simulink model "AbstractFuelControl_M3"  (R2015b)
settings: Solver=FixedStepAuto  StartTime=0.0  StopTime=simTime  RelTol=1e-3
undefined symbols (not defined in the file or in its folder): c1, c11, c12, c13, c14, c15, c16, c17, c18, c19, c2, c20, c21, c22, c23, c24, c25, c3, c4, c5, c6, c7, c8, c9, fault_time, measureTime, simTime, spec_num
settings Model: Creator=xjin  LastModifiedBy=potok
settings DataIOCC: ExternalInput=[simTime, en_speed]  LimitDataPoints=off  LoadExternalInput=on  SaveFormat=StructureWithTime  SaveOutput=off  SaveTime=off
settings DebuggingCC: UnderspecifiedInitializationDetection=Classic  MergeDetectMultiDrivingBlocksExec=none  SolverPrmCheckMsg=warning  MultiTaskRateTransMsg=warning
settings HardwareCC: ProdBitPerPointer=32  ProdLargestAtomicFloat=None  ProdIntDivRoundTo=Undefined  ProdEndianess=Unspecified  ProdWordSize=32  ProdHWDeviceType=32-bit Generic
settings GRTTargetCC: GeneratePreprocessorConditionals=Disable all
settings ConfigComp: CovModelRefEnable=Off

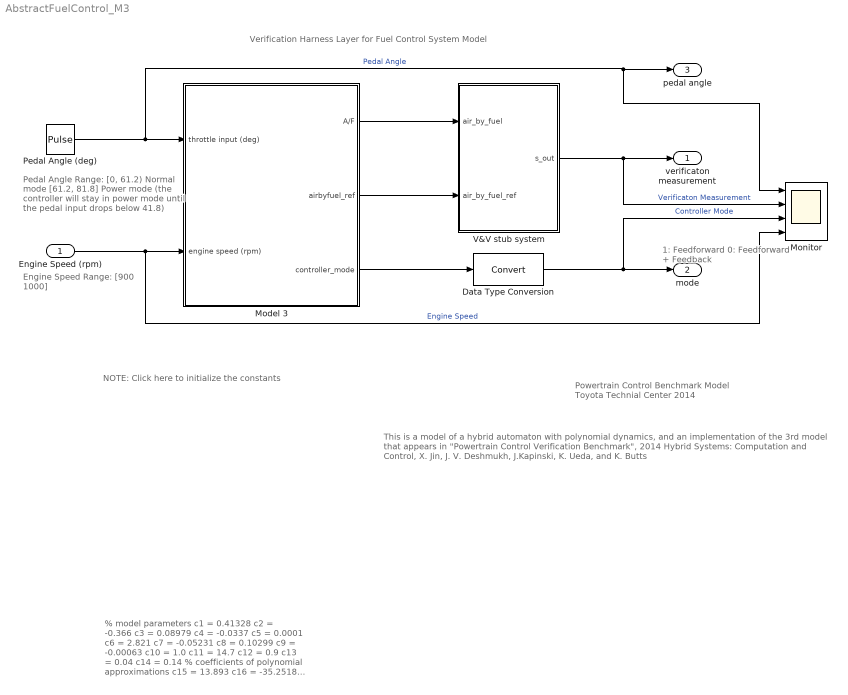
== system AbstractFuelControl_M3 ==
  note: % model parameters
      |     c1 = 0.41328
      |     c2 = -0.366
      |     c3 = 0.08979
      |     c4 = -0.0337
      |     c5 = 0.0001
      |     c6 = 2.821
      |     c7 = -0.05231
      |     c8 = 0.10299
      |     c9 = -0.00063
      |     c10 = 1.0
      |     c11 = 14.7
      |     c12 = 0.9
      |     c13 = 0.04
      |     c14 = 0.14
      | % coefficients of polynomial approximations
      |     c15 = 13.893
      |     c16 = -35.2518
      |     c17 = 20.7364
      |     c18 = 2.6287
      |     c19 = -1.592
      |     c20 = -2.3421
      |     c21 = 2.7799
      |     c22 = -0.3273
      | % sensors and actuatorerror factor
      |     c23 = 1.0
      |     c24 = 1.0
      |     c25 = 1.0
      | % simulation time
      |     simTime = 50
      | % engine speed
      |     en_speed = 1000
      | % time to start measurement for verificaiton
      |     measureTime = 1
      | % time to introduce sensor failure
      |     fault_time = 60
      | % measurement method
      |     spec_num = 1
  note: Verification Harness Layer for Fuel Control System Model
  note: 1: Feedforward
      | 0: Feedforward + Feedback
  note: Pedal Angle Range:
      | [0, 61.2) Normal mode
      | [61.2, 81.8] Power mode (the controller will
      |                    stay in power mode until the pedal
      |                    input drops below 41.8)
  note: This is a model of a hybrid automaton with polynomial dynamics, and an implementation of the 3rd model that appears in
      | "Powertrain Control Verification Benchmark", 2014 Hybrid Systems: Computation and Control,
      | X. Jin, J. V. Deshmukh, J.Kapinski, K. Ueda, and K. Butts
  note: Engine Speed Range:
      | [900 1000]
  note: Powertrain Control Benchmark Model
      | Toyota Technial Center
      | 2014
  note: NOTE: Click here to initialize the constants
  Engine Speed (rpm) : Inport
  Data Type Conversion : DataTypeConversion
  Model 3 : Subsystem  Priority=1  TreatAsAtomicUnit=on
  "Monitor " : Scope  NumInputPorts=4
  Pedal Angle (deg) : DiscretePulseGenerator  PulseType=Time based  Amplitude=53.468  Period=20.5223  PulseWidth=50  PhaseDelay=3
  V&V stub system : Subsystem  TreatAsAtomicUnit=on
  verificaton measurement : Outport
  mode : Outport  Port=2
  pedal angle : Outport  Port=3
  wires:
  V&V stub system/1("s_out ") -> "Monitor "/2, verificaton measurement/1  "Verificaton Measurement"
  Model 3/1(A/F) -> V&V stub system/1("air_by_fuel ")
  Engine Speed (rpm)/1 -> Model 3/2(engine speed (rpm)), "Monitor "/4  "Engine Speed"
  Pedal Angle (deg)/1 -> Model 3/1(throttle input (deg)), "Monitor "/1, pedal angle/1  "Pedal Angle"
  Data Type Conversion/1 -> "Monitor "/3, mode/1  "Controller Mode"
  Model 3/2(airbyfuel_ref) -> V&V stub system/2(air_by_fuel_ref)
  Model 3/3(controller_mode) -> Data Type Conversion/1

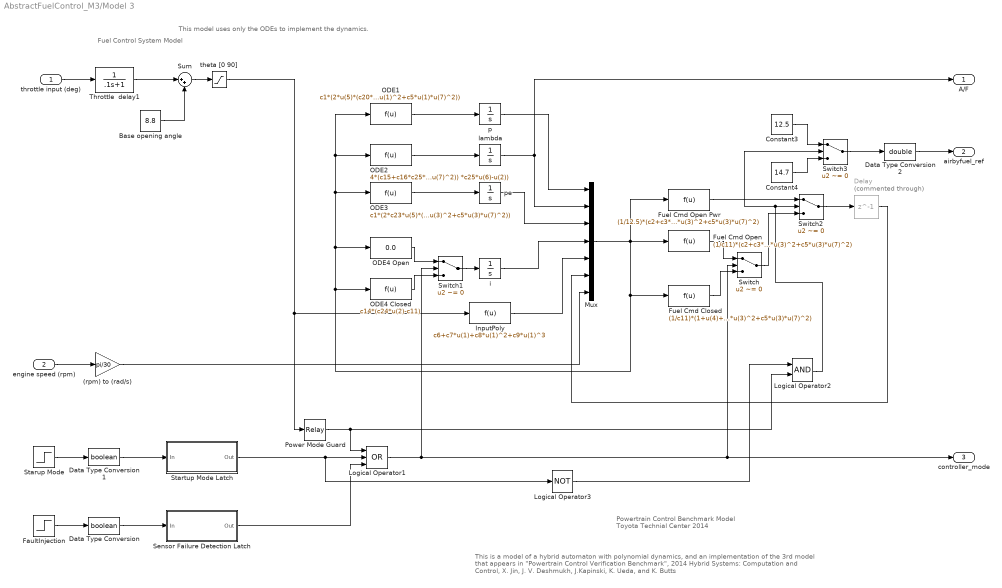
== system AbstractFuelControl_M3/Model 3 ==
  note: This model uses only the ODEs to implement the dynamics.
  note: Fuel Control System Model
  note: This is a model of a hybrid automaton with polynomial dynamics, and an implementation of the 3rd model that appears in
      | "Powertrain Control Verification Benchmark", 2014 Hybrid Systems: Computation and Control,
      | X. Jin, J. V. Deshmukh, J.Kapinski, K. Ueda, and K. Butts
  note: Powertrain Control Benchmark Model
      | Toyota Technial Center
      | 2014
  throttle input (deg) : Inport  Description=[0, 81.2]
      settings: AttributesFormatString=%<Description>
  engine speed (rpm) : Inport  Description=[900,1100]  Port=2
      settings: AttributesFormatString=%<Description>
  (rpm) to (rad/s) : Gain  Gain=pi/30
  Base opening angle : Constant  Value=8.8
  Constant3 : Constant  Value=12.5
  Constant4 : Constant  Value=14.7
  Data Type Conversion : DataTypeConversion  OutDataTypeStr=boolean
  Data Type Conversion1 : DataTypeConversion  OutDataTypeStr=boolean
  Data Type Conversion2 : DataTypeConversion  OutDataTypeStr=double
  Delay : Delay  Commented=through  DelayLength=1  InitialCondition=0
  FaultInjection : Step  Time=fault_time  SampleTime=0
      settings: AttributesFormatString=1: Failure\n0: Normal
  Fuel Cmd Closed : Fcn  Expr=(1/c11)*(1+u(4)+c13*(c24*u(2)-c11))*(c2+c3*u(7)*u(3)+c4*u(7)*u(3)^2+c5*u(3)*u(7)^2)
  Fuel Cmd Open : Fcn  Expr=(1/c11)*(c2+c3*u(7)*u(3)+c4*u(7)*u(3)^2+c5*u(3)*u(7)^2)
  Fuel Cmd Open Pwr : Fcn  Expr=(1/12.5)*(c2+c3*u(7)*u(3)+c4*u(7)*u(3)^2+c5*u(3)*u(7)^2)
  InputPoly : Fcn  Expr=c6+c7*u(1)+c8*u(1)^2+c9*u(1)^3
  Logical Operator1 : Logic  Operator=OR  Inputs=3  AllPortsSameDT=off  OutDataTypeStr=boolean
  Logical Operator2 : Logic  AllPortsSameDT=off  OutDataTypeStr=boolean
  Logical Operator3 : Logic  Operator=NOT  Inputs=3  AllPortsSameDT=off  OutDataTypeStr=boolean
  Mux : Mux  Inputs=7
  ODE1 : Fcn  Expr=c1*(2*u(5)*(c20*u(1)^2+c21*u(1)+c22) - c12*(c2+c3*u(7)*u(1)+c4*u(7)*u(1)^2+c5*u(1)*u(7)^2))
  ODE2 : Fcn  Expr=4*(c15+c16*c25*u(6)+c17*c25^2*u(6)^2+c18*(c12*(c2+c3*u(7)*u(1)+c4*u(7)*u(1)^2+c5*u(1)*u(7)^2)) +c19*(c12*(c2+c3*u(7)*u(1)+c4*u(7)*u(1)^2+c5*u(1)*u(7)^2)) *c25*u(6)-u(2))
  ODE3 : Fcn  Expr=c1*(2*c23*u(5)*(c20*u(1)^2+c21*u(1)+c22)-(c2+c3*u(7)*u(3)+c4*u(7)*u(3)^2+c5*u(3)*u(7)^2))
  ODE4 Closed : Fcn  Expr=c14*(c24*u(2)-c11)
  ODE4 Open : Fcn  Expr=0.0
  Power Mode Guard : Relay  OnSwitchValue=70  OffSwitchValue=50
  Sensor Failure Detection Latch : Subsystem  TreatAsAtomicUnit=on
  Startup Mode Latch : Subsystem  TreatAsAtomicUnit=on
  Starup Mode : Step  Time=10  Before=1  After=0  SampleTime=0
  Sum : Sum  Inputs=|++
  Switch{,1..3} (4 alike) : Switch  Criteria=u2 ~= 0
  Throttle  delay1 : TransferFcn  Denominator=[.1 1]
  i : Integrator  InitialCondition=0.017
  lambda : Integrator  InitialCondition=14.7
  p : Integrator  InitialCondition=0.6353
  pe : Integrator  InitialCondition=0.5573
  theta [0 90] : Saturate  UpperLimit=90  LowerLimit=0
  A/F : Outport
  airbyfuel_ref : Outport  Port=2
  controller_mode : Outport  Port=3
  wires:
  theta [0 90]/1 -> Power Mode Guard/1, InputPoly/1
  Base opening angle/1 -> Sum/2
  ODE1/1 -> p/1
  Mux/1 -> ODE1/1, ODE2/1, ODE3/1, ODE4 Open/1, ODE4 Closed/1, Fuel Cmd Closed/1, Fuel Cmd Open/1, Fuel Cmd Open Pwr/1
  InputPoly/1 -> Mux/5
  ODE2/1 -> lambda/1
  p/1 -> Mux/1
  pe/1 -> Mux/3
  i/1 -> Mux/4
  throttle input (deg)/1 -> Throttle  delay1/1
  lambda/1 -> Mux/2, A/F/1
  Fuel Cmd Open/1 -> Switch/1
  Fuel Cmd Closed/1 -> Switch/3
  Switch1/1 -> i/1
  ODE4 Open/1 -> Switch1/1
  ODE4 Closed/1 -> Switch1/3
  Logical Operator1/1 -> Switch1/2, controller_mode/1, Switch/2
  ODE3/1 -> pe/1
  Startup Mode Latch/1(Out) -> Logical Operator3/1, Logical Operator1/2
  Sensor Failure Detection Latch/1(Out) -> Logical Operator1/3
  Switch/1 -> Switch2/3
  Delay/1 -> Mux/6
  engine speed (rpm)/1 -> (rpm) to (rad/s)/1
  (rpm) to (rad/s)/1 -> Mux/7
  Power Mode Guard/1 -> Logical Operator2/2, Logical Operator1/1
  Fuel Cmd Open Pwr/1 -> Switch2/1
  Logical Operator3/1 -> Logical Operator2/1
  Throttle  delay1/1 -> Sum/1
  Sum/1 -> theta [0 90]/1
  Data Type Conversion/1 -> Sensor Failure Detection Latch/1(In)
  Data Type Conversion1/1 -> Startup Mode Latch/1(In)
  Starup Mode/1 -> Data Type Conversion1/1
  FaultInjection/1 -> Data Type Conversion/1
  Switch3/1 -> Data Type Conversion2/1
  Constant3/1 -> Switch3/1
  Constant4/1 -> Switch3/3
  Data Type Conversion2/1 -> airbyfuel_ref/1
  Logical Operator2/1 -> Switch2/2, Switch3/2
  Switch2/1 -> Delay/1

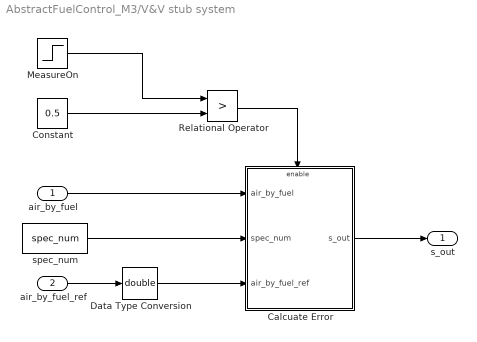
== system AbstractFuelControl_M3/V&V stub system ==
  "air_by_fuel " : Inport  OutDataTypeStr=double
  air_by_fuel_ref : Inport  Port=2
  Calcuate Error : Subsystem  Priority=20  TreatAsAtomicUnit=on
  Constant : Constant  Value=0.5
  Data Type Conversion : DataTypeConversion  OutDataTypeStr=double
  MeasureOn : Step  Time=measureTime  SampleTime=0
  Relational Operator : RelationalOperator  Operator=>  OutDataTypeStr=boolean
  spec_num : Constant  Value=spec_num  OutDataTypeStr=uint8
  "s_out " : Outport
  wires:
  Calcuate Error/1("s_out ") -> "s_out "/1
  MeasureOn/1 -> Relational Operator/1
  Constant/1 -> Relational Operator/2
  Relational Operator/1 -> Calcuate Error/Enable
  spec_num/1 -> Calcuate Error/2(spec_num)
  "air_by_fuel "/1 -> Calcuate Error/1("air_by_fuel ")
  air_by_fuel_ref/1 -> Data Type Conversion/1
  Data Type Conversion/1 -> Calcuate Error/3(air_by_fuel_ref)

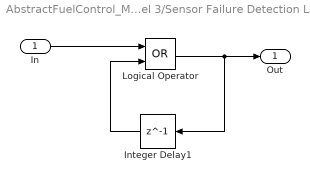
== system AbstractFuelControl_M3/Model 3/Sensor Failure Detection Latch ==
  In : Inport
  Integer Delay1 : Delay  DelayLength=1
  Logical Operator : Logic  Operator=OR  AllPortsSameDT=off
  Out : Outport
  wires:
  Logical Operator/1 -> Out/1, Integer Delay1/1
  Integer Delay1/1 -> Logical Operator/2
  In/1 -> Logical Operator/1

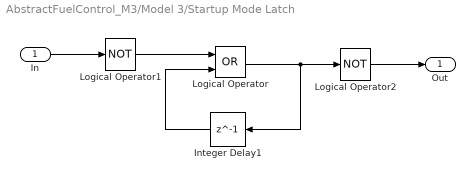
== system AbstractFuelControl_M3/Model 3/Startup Mode Latch ==
  In : Inport
  Integer Delay1 : Delay  DelayLength=1
  Logical Operator : Logic  Operator=OR  AllPortsSameDT=off
  Logical Operator1 : Logic  Operator=NOT  AllPortsSameDT=off
  Logical Operator2 : Logic  Operator=NOT  AllPortsSameDT=off
  Out : Outport
  wires:
  In/1 -> Logical Operator1/1
  Integer Delay1/1 -> Logical Operator/2
  Logical Operator/1 -> Integer Delay1/1, Logical Operator2/1
  Logical Operator1/1 -> Logical Operator/1
  Logical Operator2/1 -> Out/1

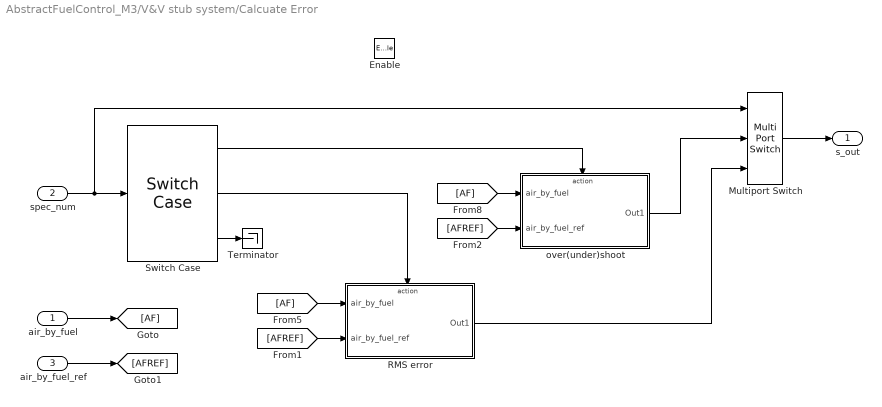
== system AbstractFuelControl_M3/V&V stub system/Calcuate Error ==
  "air_by_fuel " : Inport
  spec_num : Inport  Port=2  OutDataTypeStr=uint8
  air_by_fuel_ref : Inport  Port=3
  Enable : EnablePort
  Multiport Switch : MultiPortSwitch  Inputs=2
  RMS error : Subsystem  TreatAsAtomicUnit=on
  Switch Case : SwitchCase  CaseConditions={1,2}
  Terminator : Terminator
  over(under)shoot : Subsystem  TreatAsAtomicUnit=on
  "s_out " : Outport
  wires:
  "air_by_fuel "/1 -> [AF]
  spec_num/1 -> Multiport Switch/1, Switch Case/1
  Switch Case/1 -> over(under)shoot/Action
  [AF] -> over(under)shoot/1("air_by_fuel ")
  Switch Case/2 -> RMS error/Action
  [AF] -> RMS error/1("air_by_fuel ")
  Multiport Switch/1 -> "s_out "/1
  over(under)shoot/1(Out1) -> Multiport Switch/2
  RMS error/1(Out1) -> Multiport Switch/3
  Switch Case/3 -> Terminator/1
  air_by_fuel_ref/1 -> [AFREF]
  [AFREF] -> over(under)shoot/2(air_by_fuel_ref)
  [AFREF] -> RMS error/2(air_by_fuel_ref)

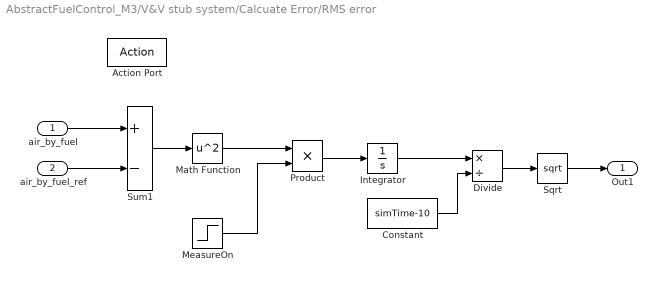
== system AbstractFuelControl_M3/V&V stub system/Calcuate Error/RMS error ==
  "air_by_fuel " : Inport
  air_by_fuel_ref : Inport  Port=2
  Action Port : ActionPort  ActionType=case
  Constant : Constant  Value=simTime-10
  Divide : Product  Inputs=*/
  Integrator : Integrator
  Math Function : Math  Operator=square  SaturateOnIntegerOverflow=on
  MeasureOn : Step  Time=10  SampleTime=0
  Product : Product
  Sqrt : Sqrt  SaturateOnIntegerOverflow=on
  Sum1 : Sum  Inputs=+-  OutDataTypeStr=Inherit: Inherit via back propagation  RndMeth=Simplest  InputSameDT=on
  Out1 : Outport
  wires:
  Sum1/1 -> Math Function/1
  Math Function/1 -> Product/1
  "air_by_fuel "/1 -> Sum1/1
  Constant/1 -> Divide/2
  air_by_fuel_ref/1 -> Sum1/2
  MeasureOn/1 -> Product/2
  Product/1 -> Integrator/1
  Divide/1 -> Sqrt/1
  Sqrt/1 -> Out1/1
  Integrator/1 -> Divide/1

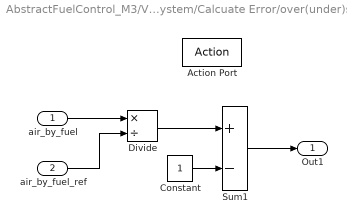
== system AbstractFuelControl_M3/V&V stub system/Calcuate Error/over(under)shoot ==
  "air_by_fuel " : Inport
  air_by_fuel_ref : Inport  Port=2
  Action Port : ActionPort  ActionType=case
  Constant : Constant
  Divide : Product  Inputs=*/
  Sum1 : Sum  Inputs=+-  OutDataTypeStr=Inherit: Inherit via back propagation  RndMeth=Simplest  InputSameDT=on
  Out1 : Outport
  wires:
  "air_by_fuel "/1 -> Divide/1
  Divide/1 -> Sum1/1
  Constant/1 -> Sum1/2
  Sum1/1 -> Out1/1
  air_by_fuel_ref/1 -> Divide/2
